simulink model "DR18E_Testpult"  (R2017a)
settings: Solver=ode1  StartTime=0.0  StopTime=Inf  FixedStep=0.001  RelTol=1e-3
PostLoadFcn:
  | , if any(exist('dsrtsu_mdlpostloadfcn', 'file') == [2, 3, 6]), try dsrtsu_mdlpostloadfcn('Execute', bdroot); catch fprintf('Error in PostLoadFcn (dsrtsu_mdlpostloadfcn) for model "%s":\n %s\n', bdroot, lasterr); end, end,
model workspace: external: MATLAB File C:\Users\DeltaRacing\Documents\dSPACE\MABX_DR18E\Model\DR18E_MABX_Parameter.m (data not in the file)
values from neighbouring files (symbols this model uses):
  am = 1/Ts    (= 1)    [DR18E_MABX_Parameter.m]
  bm = K/Ts    (= 0.05)    [DR18E_MABX_Parameter.m]
  cf = 41350    [DR18E_MABX_Parameter.m]
  cr = 41350    [DR18E_MABX_Parameter.m]
  Derating_HV_Battery_Kapa = 1    [DR18E_MABX_Parameter.m]
  Derating_Start_km = 16    [DR18E_MABX_Parameter.m]
  Drive_Mode = 0    [DR18E_MABX_Parameter.m]
  g = 1    [DR18E_MABX_Parameter.m]
  Gas_Modus = 2    [DR18E_MABX_Parameter.m]
  HV_Power_max = 80    [DR18E_MABX_Parameter.m]
  i_Getriebe = 3.3    [DR18E_MABX_Parameter.m]
  i_Lenkgetriebe = 4.32    [DR18E_MABX_Parameter.m]
  K_SET = 1    [DR18E_MABX_Parameter.m]
  Kapazitaet_HV_Battery_kWh = 6.6    [DR18E_MABX_Parameter.m]
  KW_T_Soll = 37    [DR18E_MABX_Parameter.m]
  lf = 1.2    [DR18E_MABX_Parameter.m]
  lr = 1.15    [DR18E_MABX_Parameter.m]
  m = 310    [DR18E_MABX_Parameter.m]
  M_max = 150    [DR18E_MABX_Parameter.m]
  Power_Limit_onoff = 0    [DR18E_MABX_Parameter.m]
  Reifenradius = 0.2351    [DR18E_MABX_Parameter.m]
  Strecke_Endu_km = 22    [DR18E_MABX_Parameter.m]
  TC_Decr_Gas = 0.00005    (= 5e-05)    [DR18E_MABX_Parameter.m]
  TC_Derivative = 0.4    [DR18E_MABX_Parameter.m]
  TC_Incr_Gas = 0.005    [DR18E_MABX_Parameter.m]
  TC_On = 0    [DR18E_MABX_Parameter.m]
  TC_Relay_Off = 0.065    [DR18E_MABX_Parameter.m]
  TC_Relay_On = 0.07    [DR18E_MABX_Parameter.m]
  TV_Mode = 2    [DR18E_MABX_Parameter.m]
  TV_On = 0    [DR18E_MABX_Parameter.m]
  TV_Override = 1    [DR18E_MABX_Parameter.m]
  y = 0.8    [DR18E_MABX_Parameter.m]
undefined symbols (not defined in the file or in its folder): D, DiscIntNeverNeededParam, I, K_OL, P
libraries: simulink x288, rtican x105, rtiusbflightreclib x40, rti1401lib_dio_type3 x10, simulink_extras x10, rti1401lib_adc_type4 x8, rti1401lib_II_base x7
(part 25 of 28)

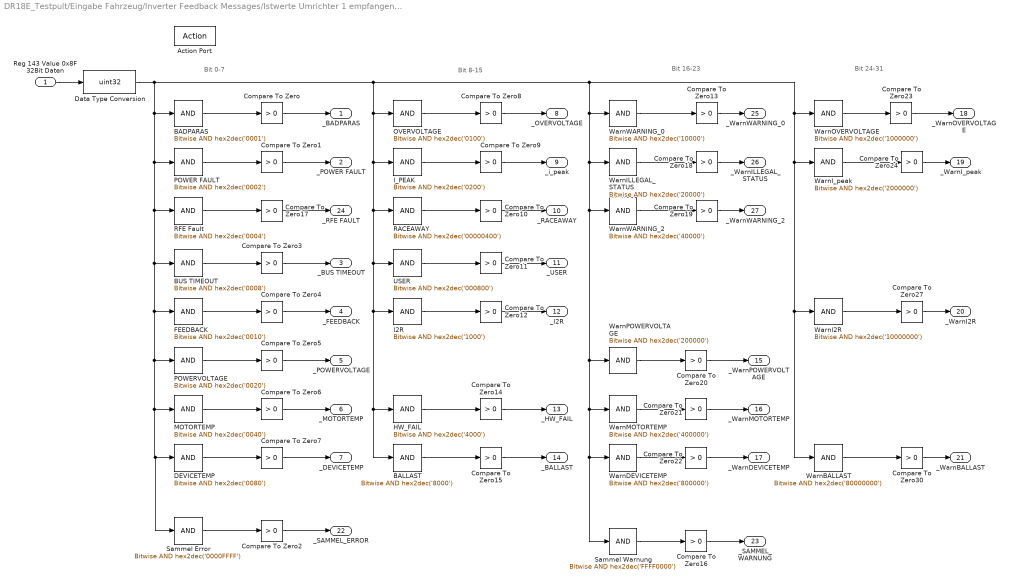
== system DR18E_Testpult/Eingabe Fahrzeug/Inverter Feedback Messages/Istwerte Umrichter 1 empfangen /Reg ID: 0x8F ERROR//Warning Register Auswertung1 ==
  note: Bit 0-7
  note: Bit 8-15
  note: Bit 16-23
  note: Bit 24-31
  Reg 143 Value 0x8F 32Bit Daten : Inport
  Action Port : ActionPort  ActionType=case
  BADPARAS : simulink/Logic and Bit Operations/Bitwise Operator  logicop=AND  UseBitMask=on  BitMask=hex2dec('0001')  BitMaskRealWorld=Stored Integer
  BALLAST : simulink/Logic and Bit Operations/Bitwise Operator  logicop=AND  UseBitMask=on  BitMask=hex2dec('8000')  BitMaskRealWorld=Stored Integer
  BUS TIMEOUT : simulink/Logic and Bit Operations/Bitwise Operator  logicop=AND  UseBitMask=on  BitMask=hex2dec('0008')  BitMaskRealWorld=Stored Integer
  Compare To Zero{,1..24,27,30} (27 alike) : simulink/Logic and Bit Operations/Compare To Zero  relop=>  OutDataTypeStr=boolean
  DEVICETEMP : simulink/Logic and Bit Operations/Bitwise Operator  logicop=AND  UseBitMask=on  BitMask=hex2dec('0080')  BitMaskRealWorld=Stored Integer
  Data Type Conversion : DataTypeConversion  OutDataTypeStr=uint32
  FEEDBACK : simulink/Logic and Bit Operations/Bitwise Operator  logicop=AND  UseBitMask=on  BitMask=hex2dec('0010')  BitMaskRealWorld=Stored Integer
  HW_FAIL : simulink/Logic and Bit Operations/Bitwise Operator  logicop=AND  UseBitMask=on  BitMask=hex2dec('4000')  BitMaskRealWorld=Stored Integer
  I2R : simulink/Logic and Bit Operations/Bitwise Operator  logicop=AND  UseBitMask=on  BitMask=hex2dec('1000')  BitMaskRealWorld=Stored Integer
  I_PEAK : simulink/Logic and Bit Operations/Bitwise Operator  logicop=AND  UseBitMask=on  BitMask=hex2dec('0200')  BitMaskRealWorld=Stored Integer
  MOTORTEMP : simulink/Logic and Bit Operations/Bitwise Operator  logicop=AND  UseBitMask=on  BitMask=hex2dec('0040')  BitMaskRealWorld=Stored Integer
  OVERVOLTAGE : simulink/Logic and Bit Operations/Bitwise Operator  logicop=AND  UseBitMask=on  BitMask=hex2dec('0100')  BitMaskRealWorld=Stored Integer
  POWER FAULT : simulink/Logic and Bit Operations/Bitwise Operator  logicop=AND  UseBitMask=on  BitMask=hex2dec('0002')  BitMaskRealWorld=Stored Integer
  POWERVOLTAGE : simulink/Logic and Bit Operations/Bitwise Operator  logicop=AND  UseBitMask=on  BitMask=hex2dec('0020')  BitMaskRealWorld=Stored Integer
  RACEAWAY : simulink/Logic and Bit Operations/Bitwise Operator  logicop=AND  UseBitMask=on  BitMask=hex2dec('00000400')  BitMaskRealWorld=Stored Integer
  RFE Fault : simulink/Logic and Bit Operations/Bitwise Operator  logicop=AND  UseBitMask=on  BitMask=hex2dec('0004')  BitMaskRealWorld=Stored Integer
  Sammel Error : simulink/Logic and Bit Operations/Bitwise Operator  logicop=AND  UseBitMask=on  BitMask=hex2dec('0000FFFF')  BitMaskRealWorld=Stored Integer
  Sammel Warnung : simulink/Logic and Bit Operations/Bitwise Operator  logicop=AND  UseBitMask=on  BitMask=hex2dec('FFFF0000')  BitMaskRealWorld=Stored Integer
  USER : simulink/Logic and Bit Operations/Bitwise Operator  logicop=AND  UseBitMask=on  BitMask=hex2dec('000800')  BitMaskRealWorld=Stored Integer
  WarnBALLAST : simulink/Logic and Bit Operations/Bitwise Operator  logicop=AND  UseBitMask=on  BitMask=hex2dec('80000000')  BitMaskRealWorld=Stored Integer
  WarnDEVICETEMP : simulink/Logic and Bit Operations/Bitwise Operator  logicop=AND  UseBitMask=on  BitMask=hex2dec('800000')  BitMaskRealWorld=Stored Integer
  WarnI2R : simulink/Logic and Bit Operations/Bitwise Operator  logicop=AND  UseBitMask=on  BitMask=hex2dec('10000000')  BitMaskRealWorld=Stored Integer
  WarnILLEGAL_STATUS : simulink/Logic and Bit Operations/Bitwise Operator  logicop=AND  UseBitMask=on  BitMask=hex2dec('20000')  BitMaskRealWorld=Stored Integer
  WarnI_peak : simulink/Logic and Bit Operations/Bitwise Operator  logicop=AND  UseBitMask=on  BitMask=hex2dec('2000000')  BitMaskRealWorld=Stored Integer
  WarnMOTORTEMP : simulink/Logic and Bit Operations/Bitwise Operator  logicop=AND  UseBitMask=on  BitMask=hex2dec('400000')  BitMaskRealWorld=Stored Integer
  WarnOVERVOLTAGE : simulink/Logic and Bit Operations/Bitwise Operator  logicop=AND  UseBitMask=on  BitMask=hex2dec('1000000')  BitMaskRealWorld=Stored Integer
  WarnPOWERVOLTAGE : simulink/Logic and Bit Operations/Bitwise Operator  logicop=AND  UseBitMask=on  BitMask=hex2dec('200000')  BitMaskRealWorld=Stored Integer
  WarnWARNING_0 : simulink/Logic and Bit Operations/Bitwise Operator  logicop=AND  UseBitMask=on  BitMask=hex2dec('10000')  BitMaskRealWorld=Stored Integer
  WarnWARNING_2 : simulink/Logic and Bit Operations/Bitwise Operator  logicop=AND  UseBitMask=on  BitMask=hex2dec('40000')  BitMaskRealWorld=Stored Integer
  _BADPARAS : Outport
  _POWER FAULT : Outport  Port=2
  _BUS TIMEOUT : Outport  Port=3
  _FEEDBACK : Outport  Port=4
  _POWERVOLTAGE : Outport  Port=5
  _MOTORTEMP : Outport  Port=6
  _DEVICETEMP : Outport  Port=7
  _OVERVOLTAGE : Outport  Port=8
  _i_peak : Outport  Port=9
  _RACEAWAY : Outport  Port=10
  _USER : Outport  Port=11
  _I2R : Outport  Port=12
  _HW_FAIL : Outport  Port=13
  _BALLAST : Outport  Port=14
  _WarnPOWERVOLTAGE : Outport  Port=15
  _WarnMOTORTEMP : Outport  Port=16
  _WarnDEVICETEMP : Outport  Port=17
  _WarnOVERVOLTAGE : Outport  Port=18
  _WarnI_peak : Outport  Port=19
  _WarnI2R : Outport  Port=20
  _WarnBALLAST : Outport  Port=21
  _SAMMEL_ERROR : Outport  Port=22
  _SAMMEL_WARNUNG : Outport  Port=23
  _RFE FAULT : Outport  Port=24
  _WarnWARNING_0 : Outport  Port=25
  _WarnILLEGAL_STATUS : Outport  Port=26
  _WarnWARNING_2 : Outport  Port=27
  wires:
  Compare To Zero16/1 -> _SAMMEL_WARNUNG/1
  Sammel Warnung/1 -> Compare To Zero16/1
  Compare To Zero2/1 -> _SAMMEL_ERROR/1
  Sammel Error/1 -> Compare To Zero2/1
  Compare To Zero30/1 -> _WarnBALLAST/1
  Compare To Zero27/1 -> _WarnI2R/1
  Reg 143 Value 0x8F 32Bit Daten/1 -> Data Type Conversion/1
  WarnBALLAST/1 -> Compare To Zero30/1
  WarnI2R/1 -> Compare To Zero27/1
  Compare To Zero24/1 -> _WarnI_peak/1
  WarnI_peak/1 -> Compare To Zero24/1
  Compare To Zero23/1 -> _WarnOVERVOLTAGE/1
  Compare To Zero22/1 -> _WarnDEVICETEMP/1
  Compare To Zero21/1 -> _WarnMOTORTEMP/1
  Compare To Zero20/1 -> _WarnPOWERVOLTAGE/1
  WarnOVERVOLTAGE/1 -> Compare To Zero23/1
  WarnDEVICETEMP/1 -> Compare To Zero22/1
  WarnMOTORTEMP/1 -> Compare To Zero21/1
  WarnPOWERVOLTAGE/1 -> Compare To Zero20/1
  Compare To Zero15/1 -> _BALLAST/1
  Compare To Zero14/1 -> _HW_FAIL/1
  Compare To Zero12/1 -> _I2R/1
  Compare To Zero11/1 -> _USER/1
  Compare To Zero10/1 -> _RACEAWAY/1
  Compare To Zero9/1 -> _i_peak/1
  Compare To Zero8/1 -> _OVERVOLTAGE/1
  BALLAST/1 -> Compare To Zero15/1
  HW_FAIL/1 -> Compare To Zero14/1
  I2R/1 -> Compare To Zero12/1
  USER/1 -> Compare To Zero11/1
  RACEAWAY/1 -> Compare To Zero10/1
  I_PEAK/1 -> Compare To Zero9/1
  OVERVOLTAGE/1 -> Compare To Zero8/1
  Compare To Zero7/1 -> _DEVICETEMP/1
  Compare To Zero6/1 -> _MOTORTEMP/1
  Compare To Zero5/1 -> _POWERVOLTAGE/1
  Compare To Zero4/1 -> _FEEDBACK/1
  Compare To Zero3/1 -> _BUS TIMEOUT/1
  Compare To Zero1/1 -> _POWER FAULT/1
  Compare To Zero/1 -> _BADPARAS/1
  DEVICETEMP/1 -> Compare To Zero7/1
  MOTORTEMP/1 -> Compare To Zero6/1
  POWERVOLTAGE/1 -> Compare To Zero5/1
  FEEDBACK/1 -> Compare To Zero4/1
  BUS TIMEOUT/1 -> Compare To Zero3/1
  POWER FAULT/1 -> Compare To Zero1/1
  BADPARAS/1 -> Compare To Zero/1
  Compare To Zero17/1 -> _RFE FAULT/1
  Data Type Conversion/1 -> BADPARAS/1, RFE Fault/1, BUS TIMEOUT/1, FEEDBACK/1, POWERVOLTAGE/1, MOTORTEMP/1, DEVICETEMP/1, Sammel Error/1, POWER FAULT/1, OVERVOLTAGE/1, RACEAWAY/1, USER/1, I2R/1, HW_FAIL/1, BALLAST/1, I_PEAK/1, WarnWARNING_0/1, WarnILLEGAL_STATUS/1, WarnWARNING_2/1, WarnMOTORTEMP/1, WarnDEVICETEMP/1, Sammel Warnung/1, WarnPOWERVOLTAGE/1, WarnOVERVOLTAGE/1, WarnI_peak/1, WarnI2R/1, WarnBALLAST/1
  RFE Fault/1 -> Compare To Zero17/1
  Compare To Zero13/1 -> _WarnWARNING_0/1
  WarnWARNING_0/1 -> Compare To Zero13/1
  Compare To Zero18/1 -> _WarnILLEGAL_STATUS/1
  WarnILLEGAL_STATUS/1 -> Compare To Zero18/1
  Compare To Zero19/1 -> _WarnWARNING_2/1
  WarnWARNING_2/1 -> Compare To Zero19/1

== system DR18E_Testpult/Eingabe Fahrzeug/Inverter Feedback Messages/Istwerte Umrichter 1 empfangen /Sender OK Detection ==
  note: This subsystem implements the surveying of the sender corresponding to the RX message.
      |
      | If for 6 consecutive execution steps no message is received it is considered that the sender is no
      | longer alive or in serious trouble and the 'RX Warn' output is set to 1.
      |
      | Also, the message is expected to be received every 50 ms approximatively. If this condition is not
      | met 6 times consecutively the 'RX Warn' output is set to 1.
  RX status : Inport
  RX delta time : Inport  Port=2
  AND : Logic
  Delta time limit : Constant  Value=0.055
  Delta time limit exceeded : RelationalOperator  RndMeth=Nearest  InputSameDT=on
  Mem{1..5} (5 alike) : Memory
  New data : RelationalOperator  Operator===  RndMeth=Nearest  InputSameDT=on
  New data value : Constant
  No data : RelationalOperator  Operator===  RndMeth=Nearest  InputSameDT=on
  No data value : Constant  Value=0
  OR : Logic  Operator=OR
  Warn : Logic  Inputs=6
  RX Warn : Outport
  wires:
  New data value/1 -> New data/2
  Delta time limit exceeded/1 -> AND/2
  Delta time limit/1 -> Delta time limit exceeded/2
  RX delta time/1 -> Delta time limit exceeded/1
  New data/1 -> AND/1
  AND/1 -> OR/2
  No data value/1 -> No data/2
  No data/1 -> OR/1
  RX status/1 -> No data/1, New data/1
  OR/1 -> Mem1/1, Warn/1
  Mem1/1 -> Mem2/1, Warn/2
  Mem2/1 -> Mem3/1, Warn/3
  Mem3/1 -> Mem4/1, Warn/4
  Warn/1 -> RX Warn/1
  Mem4/1 -> Mem5/1, Warn/5
  Mem5/1 -> Warn/6

== system DR18E_Testpult/Eingabe Fahrzeug/Inverter Feedback Messages/Istwerte Umrichter 1 empfangen /Strom ==
  In2 : Inport
  Action Port : ActionPort  ActionType=case
  Constant2 : Constant  Value=560
  Data Type Conversion4 : DataTypeConversion  OutDataTypeStr=int16
  Divide2 : Product  Inputs=*/
  Drehmoment / Strangstrom in Nm/Arms : Gain  Gain=0.75
  Gain2 : Gain  Gain=200
  Strangstrom I_rms in A U1 : Outport
  Drehmoment M in Nm U1 : Outport  Port=2
  wires:
  In2/1 -> Data Type Conversion4/1
  Gain2/1 -> Divide2/1
  Constant2/1 -> Divide2/2
  Drehmoment / Strangstrom in Nm/Arms/1 -> Drehmoment M in Nm U1/1
  Data Type Conversion4/1 -> Gain2/1
  Divide2/1 -> Drehmoment / Strangstrom in Nm/Arms/1, Strangstrom I_rms in A U1/1

== system DR18E_Testpult/Eingabe Fahrzeug/Inverter Feedback Messages/Istwerte Umrichter 1 empfangen /U_DC ==
  In1 : Inport
  Action Port : ActionPort  ActionType=case
  Umrechnung Register--> Spannung Manual BAMOCAR PG D3 S. 47 : Gain  Gain=1/31.499
  U_DC : Outport
  wires:
  In1/1 -> Umrechnung Register--> Spannung Manual BAMOCAR PG D3 S. 47/1  "Wert"
  Umrechnung Register--> Spannung Manual BAMOCAR PG D3 S. 47/1 -> U_DC/1

== system DR18E_Testpult/Eingabe Fahrzeug/Inverter Feedback Messages/Istwerte Umrichter 1 empfangen /Wirkstrom Iq ==
  In1 : Inport
  Action Port : ActionPort  ActionType=case
  Constant2 : Constant  Value=560
  Data Type Conversion1 : DataTypeConversion  OutDataTypeStr=int16
  Divide2 : Product  Inputs=*/
  Faktor 3/2 : Constant  Value=1.5
  Gain3 : Gain  Gain=200
  Polpaarzahl p : Constant  Value=10
  Product : Product  Inputs=4
  magnertischer Fluß Psi in Vs : Constant  Value=0.053
  Wirkstrom Iq in A U1 : Outport
  Drehmoment in Nm aus Iq U1 : Outport  Port=2
  wires:
  Divide2/1 -> Wirkstrom Iq in A U1/1, Product/1
  In1/1 -> Data Type Conversion1/1
  Gain3/1 -> Divide2/1
  Constant2/1 -> Divide2/2
  Polpaarzahl p/1 -> Product/2
  Faktor 3/2/1 -> Product/3
  magnertischer Fluß Psi in Vs/1 -> Product/4
  Product/1 -> Drehmoment in Nm aus Iq U1/1
  Data Type Conversion1/1 -> Gain3/1

== system DR18E_Testpult/Eingabe Fahrzeug/Inverter Feedback Messages/Istwerte Umrichter 2 empfangen/Drehzahl ==
  CAN Value : Inport
  M_Mot : Inport  Port=2
  Action Port : ActionPort  ActionType=case
  2*p / 60i : Gain  Gain=1.8*6.283185 / 60
  Constant1 : Constant  Value=-1
  Data Type Conversion : DataTypeConversion  OutDataTypeStr=int16
  Data Type Conversion1 : DataTypeConversion  OutDataTypeStr=double
  PT1 Discrete2 : Subsystem
  Product : Product
  Skalierung Drehzahl : Subsystem  TreatAsAtomicUnit=on
  TFilterDrehzahl : Constant  Value=0.01
  Drehzahl in 1/min U1 : Outport
  Motorleistung in W U1 : Outport  Port=2
  wires:
  CAN Value/1 -> Data Type Conversion/1
  PT1 Discrete2/1(y) -> Drehzahl in 1/min U1/1, Product/1
  Data Type Conversion/1 -> Data Type Conversion1/1
  Product/1 -> 2*p / 60i/1
  M_Mot/1 -> Product/2
  2*p / 60i/1 -> Motorleistung in W U1/1
  Constant1/1 -> PT1 Discrete2/2(K)
  TFilterDrehzahl/1 -> PT1 Discrete2/3(T)
  Skalierung Drehzahl/1(Out1) -> PT1 Discrete2/1(u)
  Data Type Conversion1/1 -> Skalierung Drehzahl/1(In1)

== system DR18E_Testpult/Eingabe Fahrzeug/Inverter Feedback Messages/Istwerte Umrichter 2 empfangen/FlightRecorder2 ==
  In1 : Inport
  Data Type Conversion : DataTypeConversion
  Gain : Gain
  USB_FLIGHT_REC_BL1 : rtiusbflightreclib/USB_FLIGHT_REC_BL1  VarName=MMotR_Ist  DataType=Single  SampleTime=-1  TLCFileName=rtiusbflightrecwrite  Reserved1=[]  Reserved2=[]  Reserved3=[]  Reserved4=[]  DSProperties=struct('RTI',struct('Version',uint32(3),'BlockType',struct('isSLSource',uint8(0),'isSLSink',uint8(1),'isHWSource',uint8(0),'isHWSink',uint8(0),'isSetup',uint8(0),'isInline',uint8(1),'isNonInline',uint8(0),'isInterrupt',uint8(0),'isChannelwise',uint8(0)),'IOBoardType',{{'DSUSB','FLIGHTREC'}},'UnitType','FLIGHTREC','Identifier','WRITE','DialogType','SL','BlockSet','RTIUSBFLIGHTREC','SlaveProcessor','NONE'))  RTIBlockInterface=struct('InputPortsActive',1,'InputPortsWidth',int32(1),'InputPortsDataType',{{'SS_SINGLE'}},'BlockDisplay',{{['Write to\nUSB Flight Recorder'],'center'}},'IconTransparency','off','InitLevel',3,'BlockName',struct('Token',{{'USB_FLIGHT_REC_BL1'}}),'MaskDescription',['Write input to the Flight Recorder. Recorded data can be referenced by the specified variable.'],'SampleTime',{{-1}})  RTIBlockParameters=struct('VarName',{{'MMotR_Ist','OFF',[]}},'DataType',{{'Single','OFF',[]}},'SampleTime',{{-1,'OFF',[]}},'TLCFileName',{{'rtiusbflightrecwrite','OFF',[]}})  RTISFcnParameters=struct('VarName','char','DataType','char','SampleTime','double','TLCFileName','char')  RTIBlockParaDefault=struct('VarName','Var1','DataType','Single','SampleTime',-1,'TLCFileName','rtiusbflightrecwrite')
      settings: SourceProductName=dSPACE RTI USB Flight Rec Blockset
  wires:
  Data Type Conversion/1 -> USB_FLIGHT_REC_BL1/1
  In1/1 -> Gain/1
  Gain/1 -> Data Type Conversion/1

== system DR18E_Testpult/Eingabe Fahrzeug/Inverter Feedback Messages/Istwerte Umrichter 2 empfangen/Inverter_Temp ==
  In1 : Inport
  Action Port : ActionPort  ActionType=case
  "BAMOCAR PG D3 Manual S. 48 " : Lookup_n-D  NumberOfTableDimensions=1  BreakpointsForDimension1=[17151,17400,17688,18017,18387,18797,19247,19733,20250,20793,21357,21933,22515,23097,23671,24232,24775,25296,25792,26261,26702]  Table=[0,5,10,15,20,25,30,35,40,45,50,55,60,65,70,75,80,85,90,95,100]  RndMeth=Simplest  InputSameDT=on
  Inverter_Temp : Outport
  wires:
  In1/1 -> "BAMOCAR PG D3 Manual S. 48 "/1  "Wert"
  "BAMOCAR PG D3 Manual S. 48 "/1 -> Inverter_Temp/1

== system DR18E_Testpult/Eingabe Fahrzeug/Inverter Feedback Messages/Istwerte Umrichter 2 empfangen/Motortemperatur ==
  In1 : Inport
  Action Port : ActionPort  ActionType=case
  Constant2 : Constant  Value=37175
  Divide : Product  Inputs=*/
  Gain : Gain  Gain=4700
  Subtract : Sum  Inputs=+-
  Temp. corresponding resistance : Lookup_n-D  NumberOfTableDimensions=1  BreakpointsForDimension1=[1030,1135,1247,1367,1495,1630,1772,1922,2000,2080,2245,2417,2597,2785,2980,3182,3392,3607,3817,3915,4008,4166,4280]  IndexSearchMethod=Linear search  Table=[-50,-40,-30,-20,-10,0,10,20,25,30,40,50,60,70,80,90,100,110,120,125,130,140,150]  RndMeth=Simplest  InputSameDT=on
  Motor1_Temp : Outport
  "Motor1_R " : Outport  Port=2
  wires:
  Gain/1 -> Divide/1
  Subtract/1 -> Divide/2
  Constant2/1 -> Subtract/1
  In1/1 -> Subtract/2, Gain/1  "Wert"
  Divide/1 -> "Motor1_R "/1, Temp. corresponding resistance/1
  Temp. corresponding resistance/1 -> Motor1_Temp/1

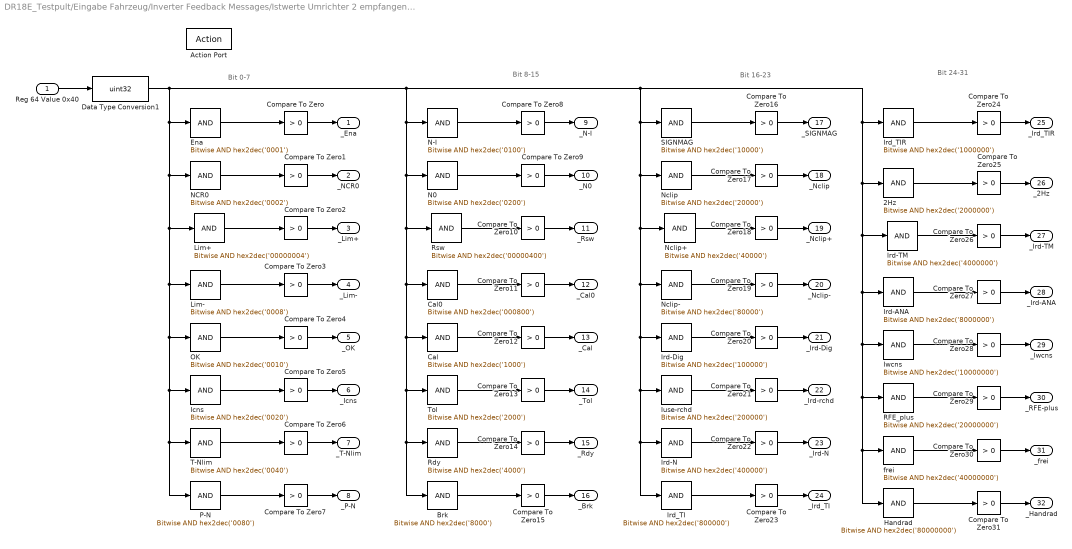
== system DR18E_Testpult/Eingabe Fahrzeug/Inverter Feedback Messages/Istwerte Umrichter 2 empfangen/Red ID 64: Status Register Auswertung ==
  note: Bit 16-23
  note: Bit 24-31
  note: Bit 8-15
  note: Bit 0-7
  Reg 64 Value 0x40 : Inport
  Action Port : ActionPort  ActionType=case
  2Hz : simulink/Logic and Bit Operations/Bitwise Operator  logicop=AND  UseBitMask=on  BitMask=hex2dec('2000000')  BitMaskRealWorld=Stored Integer
  Brk : simulink/Logic and Bit Operations/Bitwise Operator  logicop=AND  UseBitMask=on  BitMask=hex2dec('8000')  BitMaskRealWorld=Stored Integer
  Cal : simulink/Logic and Bit Operations/Bitwise Operator  logicop=AND  UseBitMask=on  BitMask=hex2dec('1000')  BitMaskRealWorld=Stored Integer
  Cal0 : simulink/Logic and Bit Operations/Bitwise Operator  logicop=AND  UseBitMask=on  BitMask=hex2dec('000800')  BitMaskRealWorld=Stored Integer
  Compare To Zero{,1..31} (32 alike) : simulink/Logic and Bit Operations/Compare To Zero  relop=>  OutDataTypeStr=boolean
  Data Type Conversion1 : DataTypeConversion  OutDataTypeStr=uint32
  Ena : simulink/Logic and Bit Operations/Bitwise Operator  logicop=AND  UseBitMask=on  BitMask=hex2dec('0001')  BitMaskRealWorld=Stored Integer
  Handrad : simulink/Logic and Bit Operations/Bitwise Operator  logicop=AND  UseBitMask=on  BitMask=hex2dec('80000000')  BitMaskRealWorld=Stored Integer
  Icns : simulink/Logic and Bit Operations/Bitwise Operator  logicop=AND  UseBitMask=on  BitMask=hex2dec('0020')  BitMaskRealWorld=Stored Integer
  Ird-ANA : simulink/Logic and Bit Operations/Bitwise Operator  logicop=AND  UseBitMask=on  BitMask=hex2dec('8000000')  BitMaskRealWorld=Stored Integer
  Ird-Dig : simulink/Logic and Bit Operations/Bitwise Operator  logicop=AND  UseBitMask=on  BitMask=hex2dec('100000')  BitMaskRealWorld=Stored Integer
  Ird-N : simulink/Logic and Bit Operations/Bitwise Operator  logicop=AND  UseBitMask=on  BitMask=hex2dec('400000')  BitMaskRealWorld=Stored Integer
  Ird-TM : simulink/Logic and Bit Operations/Bitwise Operator  logicop=AND  UseBitMask=on  BitMask=hex2dec('4000000')  BitMaskRealWorld=Stored Integer
  Ird_TI : simulink/Logic and Bit Operations/Bitwise Operator  logicop=AND  UseBitMask=on  BitMask=hex2dec('800000')  BitMaskRealWorld=Stored Integer
  Ird_TIR : simulink/Logic and Bit Operations/Bitwise Operator  logicop=AND  UseBitMask=on  BitMask=hex2dec('1000000')  BitMaskRealWorld=Stored Integer
  Iuse-rchd : simulink/Logic and Bit Operations/Bitwise Operator  logicop=AND  UseBitMask=on  BitMask=hex2dec('200000')  BitMaskRealWorld=Stored Integer
  Iwcns : simulink/Logic and Bit Operations/Bitwise Operator  logicop=AND  UseBitMask=on  BitMask=hex2dec('10000000')  BitMaskRealWorld=Stored Integer
  Lim+ : simulink/Logic and Bit Operations/Bitwise Operator  logicop=AND  UseBitMask=on  BitMask=hex2dec('00000004')  BitMaskRealWorld=Stored Integer
  Lim- : simulink/Logic and Bit Operations/Bitwise Operator  logicop=AND  UseBitMask=on  BitMask=hex2dec('0008')  BitMaskRealWorld=Stored Integer
  N-I : simulink/Logic and Bit Operations/Bitwise Operator  logicop=AND  UseBitMask=on  BitMask=hex2dec('0100')  BitMaskRealWorld=Stored Integer
  N0 : simulink/Logic and Bit Operations/Bitwise Operator  logicop=AND  UseBitMask=on  BitMask=hex2dec('0200')  BitMaskRealWorld=Stored Integer
  NCR0 : simulink/Logic and Bit Operations/Bitwise Operator  logicop=AND  UseBitMask=on  BitMask=hex2dec('0002')  BitMaskRealWorld=Stored Integer
  Nclip : simulink/Logic and Bit Operations/Bitwise Operator  logicop=AND  UseBitMask=on  BitMask=hex2dec('20000')  BitMaskRealWorld=Stored Integer
  Nclip+ : simulink/Logic and Bit Operations/Bitwise Operator  logicop=AND  UseBitMask=on  BitMask=hex2dec('40000')  BitMaskRealWorld=Stored Integer
  Nclip- : simulink/Logic and Bit Operations/Bitwise Operator  logicop=AND  UseBitMask=on  BitMask=hex2dec('80000')  BitMaskRealWorld=Stored Integer
  OK : simulink/Logic and Bit Operations/Bitwise Operator  logicop=AND  UseBitMask=on  BitMask=hex2dec('0010')  BitMaskRealWorld=Stored Integer
  P-N : simulink/Logic and Bit Operations/Bitwise Operator  logicop=AND  UseBitMask=on  BitMask=hex2dec('0080')  BitMaskRealWorld=Stored Integer
  RFE_plus : simulink/Logic and Bit Operations/Bitwise Operator  logicop=AND  UseBitMask=on  BitMask=hex2dec('20000000')  BitMaskRealWorld=Stored Integer
  Rdy : simulink/Logic and Bit Operations/Bitwise Operator  logicop=AND  UseBitMask=on  BitMask=hex2dec('4000')  BitMaskRealWorld=Stored Integer
  Rsw : simulink/Logic and Bit Operations/Bitwise Operator  logicop=AND  UseBitMask=on  BitMask=hex2dec('00000400')  BitMaskRealWorld=Stored Integer
  SIGNMAG : simulink/Logic and Bit Operations/Bitwise Operator  logicop=AND  UseBitMask=on  BitMask=hex2dec('10000')  BitMaskRealWorld=Stored Integer
  T-Nlim : simulink/Logic and Bit Operations/Bitwise Operator  logicop=AND  UseBitMask=on  BitMask=hex2dec('0040')  BitMaskRealWorld=Stored Integer
  Tol : simulink/Logic and Bit Operations/Bitwise Operator  logicop=AND  UseBitMask=on  BitMask=hex2dec('2000')  BitMaskRealWorld=Stored Integer
  frei : simulink/Logic and Bit Operations/Bitwise Operator  logicop=AND  UseBitMask=on  BitMask=hex2dec('40000000')  BitMaskRealWorld=Stored Integer
  _Ena : Outport
  _NCR0 : Outport  Port=2
  _Lim+ : Outport  Port=3
  _Lim- : Outport  Port=4
  _OK : Outport  Port=5
  _Icns : Outport  Port=6
  _T-Nlim : Outport  Port=7
  _P-N : Outport  Port=8
  _N-I : Outport  Port=9
  _N0 : Outport  Port=10
  _Rsw : Outport  Port=11
  _Cal0 : Outport  Port=12
  _Cal : Outport  Port=13
  _Tol : Outport  Port=14
  _Rdy : Outport  Port=15
  _Brk : Outport  Port=16
  _SIGNMAG : Outport  Port=17
  _Nclip : Outport  Port=18
  _Nclip+ : Outport  Port=19
  _Nclip- : Outport  Port=20
  _Ird-Dig : Outport  Port=21
  _Ird-rchd : Outport  Port=22
  _Ird-N : Outport  Port=23
  _Ird_TI : Outport  Port=24
  _Ird_TIR : Outport  Port=25
  _2Hz : Outport  Port=26
  _Ird-TM : Outport  Port=27
  _Ird-ANA : Outport  Port=28
  _Iwcns : Outport  Port=29
  _RFE-plus : Outport  Port=30
  _frei : Outport  Port=31
  _Handrad : Outport  Port=32
  wires:
  Reg 64 Value 0x40/1 -> Data Type Conversion1/1
  2Hz/1 -> Compare To Zero25/1
  Iwcns/1 -> Compare To Zero28/1
  Compare To Zero25/1 -> _2Hz/1
  Compare To Zero29/1 -> _RFE-plus/1
  Ird-ANA/1 -> Compare To Zero27/1
  Compare To Zero26/1 -> _Ird-TM/1
  Handrad/1 -> Compare To Zero31/1
  RFE_plus/1 -> Compare To Zero29/1
  Compare To Zero27/1 -> _Ird-ANA/1
  Ird-TM/1 -> Compare To Zero26/1
  frei/1 -> Compare To Zero30/1
  Compare To Zero28/1 -> _Iwcns/1
  Tol/1 -> Compare To Zero13/1
  Nclip+/1 -> Compare To Zero18/1
  Compare To Zero17/1 -> _Nclip/1
  Compare To Zero16/1 -> _SIGNMAG/1
  Ird-N/1 -> Compare To Zero22/1
  Ird_TI/1 -> Compare To Zero23/1
  Compare To Zero20/1 -> _Ird-Dig/1
  Lim+/1 -> Compare To Zero2/1
  Nclip-/1 -> Compare To Zero19/1
  SIGNMAG/1 -> Compare To Zero16/1
  Compare To Zero12/1 -> _Cal/1
  Compare To Zero3/1 -> _Lim-/1
  Compare To Zero2/1 -> _Lim+/1
  Compare To Zero8/1 -> _N-I/1
  N-I/1 -> Compare To Zero8/1
  Brk/1 -> Compare To Zero15/1
  Compare To Zero/1 -> _Ena/1
  Compare To Zero6/1 -> _T-Nlim/1
  Compare To Zero1/1 -> _NCR0/1
  P-N/1 -> Compare To Zero7/1
  Icns/1 -> Compare To Zero5/1
  T-Nlim/1 -> Compare To Zero6/1
  Compare To Zero9/1 -> _N0/1
  Cal/1 -> Compare To Zero12/1
  Rdy/1 -> Compare To Zero14/1
  Compare To Zero5/1 -> _Icns/1
  NCR0/1 -> Compare To Zero1/1
  Ena/1 -> Compare To Zero/1
  Compare To Zero30/1 -> _frei/1
  Iuse-rchd/1 -> Compare To Zero21/1
  Compare To Zero19/1 -> _Nclip-/1
  Compare To Zero23/1 -> _Ird_TI/1
  Ird_TIR/1 -> Compare To Zero24/1
  Compare To Zero31/1 -> _Handrad/1
  Cal0/1 -> Compare To Zero11/1
  Compare To Zero7/1 -> _P-N/1
  Compare To Zero24/1 -> _Ird_TIR/1
  Compare To Zero22/1 -> _Ird-N/1
  Compare To Zero4/1 -> _OK/1
  Compare To Zero10/1 -> _Rsw/1
  Compare To Zero21/1 -> _Ird-rchd/1
  Compare To Zero15/1 -> _Brk/1
  Compare To Zero11/1 -> _Cal0/1
  OK/1 -> Compare To Zero4/1
  Compare To Zero13/1 -> _Tol/1
  Compare To Zero14/1 -> _Rdy/1
  N0/1 -> Compare To Zero9/1
  Ird-Dig/1 -> Compare To Zero20/1
  Lim-/1 -> Compare To Zero3/1
  Compare To Zero18/1 -> _Nclip+/1
  Nclip/1 -> Compare To Zero17/1
  Rsw/1 -> Compare To Zero10/1
  Data Type Conversion1/1 -> 2Hz/1, Handrad/1, frei/1, RFE_plus/1, Iwcns/1, Ird-ANA/1, Ird-TM/1, Ird_TIR/1, Nclip/1, Ird_TI/1, Ird-N/1, Iuse-rchd/1, Ird-Dig/1, Nclip-/1, Nclip+/1, SIGNMAG/1, N0/1, Brk/1, Rdy/1, Tol/1, Cal/1, Cal0/1, Rsw/1, N-I/1, NCR0/1, P-N/1, T-Nlim/1, Icns/1, OK/1, Lim-/1, Lim+/1, Ena/1

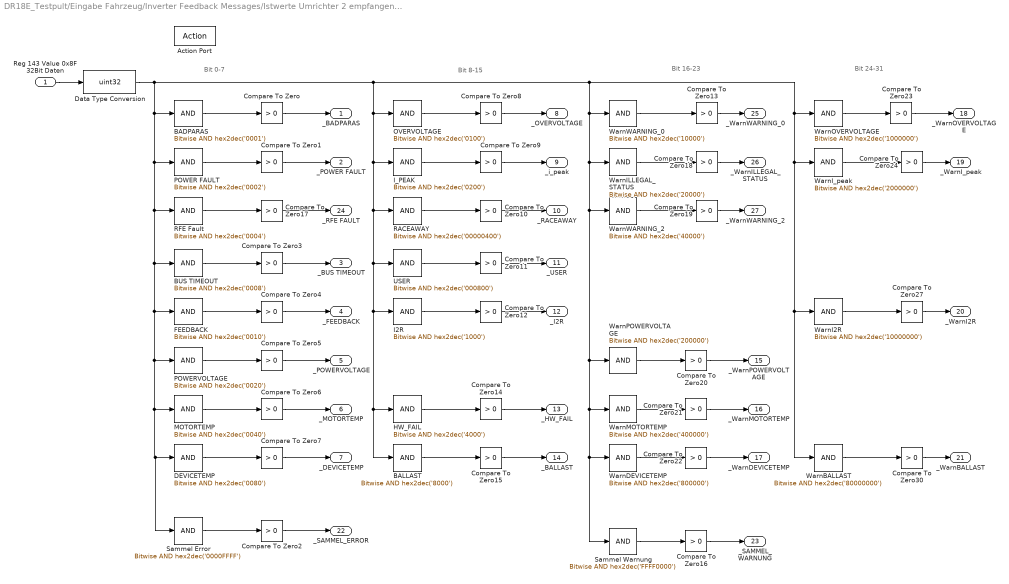
== system DR18E_Testpult/Eingabe Fahrzeug/Inverter Feedback Messages/Istwerte Umrichter 2 empfangen/Reg ID: 0x8F ERROR//Warning Register Auswertung1 ==
  note: Bit 8-15
  note: Bit 0-7
  note: Bit 24-31
  note: Bit 16-23
  Reg 143 Value 0x8F 32Bit Daten : Inport
  Action Port : ActionPort  ActionType=case
  BADPARAS : simulink/Logic and Bit Operations/Bitwise Operator  logicop=AND  UseBitMask=on  BitMask=hex2dec('0001')  BitMaskRealWorld=Stored Integer
  BALLAST : simulink/Logic and Bit Operations/Bitwise Operator  logicop=AND  UseBitMask=on  BitMask=hex2dec('8000')  BitMaskRealWorld=Stored Integer
  BUS TIMEOUT : simulink/Logic and Bit Operations/Bitwise Operator  logicop=AND  UseBitMask=on  BitMask=hex2dec('0008')  BitMaskRealWorld=Stored Integer
  Compare To Zero{,1..24,27,30} (27 alike) : simulink/Logic and Bit Operations/Compare To Zero  relop=>  OutDataTypeStr=boolean
  DEVICETEMP : simulink/Logic and Bit Operations/Bitwise Operator  logicop=AND  UseBitMask=on  BitMask=hex2dec('0080')  BitMaskRealWorld=Stored Integer
  Data Type Conversion : DataTypeConversion  OutDataTypeStr=uint32
  FEEDBACK : simulink/Logic and Bit Operations/Bitwise Operator  logicop=AND  UseBitMask=on  BitMask=hex2dec('0010')  BitMaskRealWorld=Stored Integer
  HW_FAIL : simulink/Logic and Bit Operations/Bitwise Operator  logicop=AND  UseBitMask=on  BitMask=hex2dec('4000')  BitMaskRealWorld=Stored Integer
  I2R : simulink/Logic and Bit Operations/Bitwise Operator  logicop=AND  UseBitMask=on  BitMask=hex2dec('1000')  BitMaskRealWorld=Stored Integer
  I_PEAK : simulink/Logic and Bit Operations/Bitwise Operator  logicop=AND  UseBitMask=on  BitMask=hex2dec('0200')  BitMaskRealWorld=Stored Integer
  MOTORTEMP : simulink/Logic and Bit Operations/Bitwise Operator  logicop=AND  UseBitMask=on  BitMask=hex2dec('0040')  BitMaskRealWorld=Stored Integer
  OVERVOLTAGE : simulink/Logic and Bit Operations/Bitwise Operator  logicop=AND  UseBitMask=on  BitMask=hex2dec('0100')  BitMaskRealWorld=Stored Integer
  POWER FAULT : simulink/Logic and Bit Operations/Bitwise Operator  logicop=AND  UseBitMask=on  BitMask=hex2dec('0002')  BitMaskRealWorld=Stored Integer
  POWERVOLTAGE : simulink/Logic and Bit Operations/Bitwise Operator  logicop=AND  UseBitMask=on  BitMask=hex2dec('0020')  BitMaskRealWorld=Stored Integer
  RACEAWAY : simulink/Logic and Bit Operations/Bitwise Operator  logicop=AND  UseBitMask=on  BitMask=hex2dec('00000400')  BitMaskRealWorld=Stored Integer
  RFE Fault : simulink/Logic and Bit Operations/Bitwise Operator  logicop=AND  UseBitMask=on  BitMask=hex2dec('0004')  BitMaskRealWorld=Stored Integer
  Sammel Error : simulink/Logic and Bit Operations/Bitwise Operator  logicop=AND  UseBitMask=on  BitMask=hex2dec('0000FFFF')  BitMaskRealWorld=Stored Integer
  Sammel Warnung : simulink/Logic and Bit Operations/Bitwise Operator  logicop=AND  UseBitMask=on  BitMask=hex2dec('FFFF0000')  BitMaskRealWorld=Stored Integer
  USER : simulink/Logic and Bit Operations/Bitwise Operator  logicop=AND  UseBitMask=on  BitMask=hex2dec('000800')  BitMaskRealWorld=Stored Integer
  WarnBALLAST : simulink/Logic and Bit Operations/Bitwise Operator  logicop=AND  UseBitMask=on  BitMask=hex2dec('80000000')  BitMaskRealWorld=Stored Integer
  WarnDEVICETEMP : simulink/Logic and Bit Operations/Bitwise Operator  logicop=AND  UseBitMask=on  BitMask=hex2dec('800000')  BitMaskRealWorld=Stored Integer
  WarnI2R : simulink/Logic and Bit Operations/Bitwise Operator  logicop=AND  UseBitMask=on  BitMask=hex2dec('10000000')  BitMaskRealWorld=Stored Integer
  WarnILLEGAL_STATUS : simulink/Logic and Bit Operations/Bitwise Operator  logicop=AND  UseBitMask=on  BitMask=hex2dec('20000')  BitMaskRealWorld=Stored Integer
  WarnI_peak : simulink/Logic and Bit Operations/Bitwise Operator  logicop=AND  UseBitMask=on  BitMask=hex2dec('2000000')  BitMaskRealWorld=Stored Integer
  WarnMOTORTEMP : simulink/Logic and Bit Operations/Bitwise Operator  logicop=AND  UseBitMask=on  BitMask=hex2dec('400000')  BitMaskRealWorld=Stored Integer
  WarnOVERVOLTAGE : simulink/Logic and Bit Operations/Bitwise Operator  logicop=AND  UseBitMask=on  BitMask=hex2dec('1000000')  BitMaskRealWorld=Stored Integer
  WarnPOWERVOLTAGE : simulink/Logic and Bit Operations/Bitwise Operator  logicop=AND  UseBitMask=on  BitMask=hex2dec('200000')  BitMaskRealWorld=Stored Integer
  WarnWARNING_0 : simulink/Logic and Bit Operations/Bitwise Operator  logicop=AND  UseBitMask=on  BitMask=hex2dec('10000')  BitMaskRealWorld=Stored Integer
  WarnWARNING_2 : simulink/Logic and Bit Operations/Bitwise Operator  logicop=AND  UseBitMask=on  BitMask=hex2dec('40000')  BitMaskRealWorld=Stored Integer
  _BADPARAS : Outport
  _POWER FAULT : Outport  Port=2
  _BUS TIMEOUT : Outport  Port=3
  _FEEDBACK : Outport  Port=4
  _POWERVOLTAGE : Outport  Port=5
  _MOTORTEMP : Outport  Port=6
  _DEVICETEMP : Outport  Port=7
  _OVERVOLTAGE : Outport  Port=8
  _i_peak : Outport  Port=9
  _RACEAWAY : Outport  Port=10
  _USER : Outport  Port=11
  _I2R : Outport  Port=12
  _HW_FAIL : Outport  Port=13
  _BALLAST : Outport  Port=14
  _WarnPOWERVOLTAGE : Outport  Port=15
  _WarnMOTORTEMP : Outport  Port=16
  _WarnDEVICETEMP : Outport  Port=17
  _WarnOVERVOLTAGE : Outport  Port=18
  _WarnI_peak : Outport  Port=19
  _WarnI2R : Outport  Port=20
  _WarnBALLAST : Outport  Port=21
  _SAMMEL_ERROR : Outport  Port=22
  _SAMMEL_WARNUNG : Outport  Port=23
  _RFE FAULT : Outport  Port=24
  _WarnWARNING_0 : Outport  Port=25
  _WarnILLEGAL_STATUS : Outport  Port=26
  _WarnWARNING_2 : Outport  Port=27
  wires:
  Reg 143 Value 0x8F 32Bit Daten/1 -> Data Type Conversion/1
  MOTORTEMP/1 -> Compare To Zero6/1
  BUS TIMEOUT/1 -> Compare To Zero3/1
  Compare To Zero12/1 -> _I2R/1
  FEEDBACK/1 -> Compare To Zero4/1
  HW_FAIL/1 -> Compare To Zero14/1
  BADPARAS/1 -> Compare To Zero/1
  Compare To Zero3/1 -> _BUS TIMEOUT/1
  DEVICETEMP/1 -> Compare To Zero7/1
  Compare To Zero6/1 -> _MOTORTEMP/1
  WarnBALLAST/1 -> Compare To Zero30/1
  RACEAWAY/1 -> Compare To Zero10/1
  Compare To Zero15/1 -> _BALLAST/1
  Compare To Zero5/1 -> _POWERVOLTAGE/1
  OVERVOLTAGE/1 -> Compare To Zero8/1
  Compare To Zero1/1 -> _POWER FAULT/1
  Compare To Zero9/1 -> _i_peak/1
  Compare To Zero4/1 -> _FEEDBACK/1
  Compare To Zero/1 -> _BADPARAS/1
  Compare To Zero10/1 -> _RACEAWAY/1
  I_PEAK/1 -> Compare To Zero9/1
  BALLAST/1 -> Compare To Zero15/1
  USER/1 -> Compare To Zero11/1
  Compare To Zero14/1 -> _HW_FAIL/1
  Compare To Zero8/1 -> _OVERVOLTAGE/1
  Compare To Zero16/1 -> _SAMMEL_WARNUNG/1
  Compare To Zero23/1 -> _WarnOVERVOLTAGE/1
  Compare To Zero11/1 -> _USER/1
  WarnPOWERVOLTAGE/1 -> Compare To Zero20/1
  Compare To Zero27/1 -> _WarnI2R/1
  Compare To Zero2/1 -> _SAMMEL_ERROR/1
  WarnOVERVOLTAGE/1 -> Compare To Zero23/1
  WarnI_peak/1 -> Compare To Zero24/1
  Sammel Warnung/1 -> Compare To Zero16/1
  POWERVOLTAGE/1 -> Compare To Zero5/1
  Compare To Zero7/1 -> _DEVICETEMP/1
  WarnI2R/1 -> Compare To Zero27/1
  POWER FAULT/1 -> Compare To Zero1/1
  WarnMOTORTEMP/1 -> Compare To Zero21/1
  WarnDEVICETEMP/1 -> Compare To Zero22/1
  Compare To Zero30/1 -> _WarnBALLAST/1
  Sammel Error/1 -> Compare To Zero2/1
  RFE Fault/1 -> Compare To Zero17/1
  Compare To Zero22/1 -> _WarnDEVICETEMP/1
  Compare To Zero17/1 -> _RFE FAULT/1
  Data Type Conversion/1 -> BADPARAS/1, RFE Fault/1, BUS TIMEOUT/1, FEEDBACK/1, POWERVOLTAGE/1, MOTORTEMP/1, DEVICETEMP/1, Sammel Error/1, POWER FAULT/1, OVERVOLTAGE/1, RACEAWAY/1, USER/1, I2R/1, HW_FAIL/1, BALLAST/1, I_PEAK/1, WarnWARNING_0/1, WarnILLEGAL_STATUS/1, WarnWARNING_2/1, WarnMOTORTEMP/1, WarnDEVICETEMP/1, Sammel Warnung/1, WarnPOWERVOLTAGE/1, WarnOVERVOLTAGE/1, WarnI_peak/1, WarnI2R/1, WarnBALLAST/1
  I2R/1 -> Compare To Zero12/1
  Compare To Zero21/1 -> _WarnMOTORTEMP/1
  Compare To Zero20/1 -> _WarnPOWERVOLTAGE/1
  Compare To Zero19/1 -> _WarnWARNING_2/1
  Compare To Zero18/1 -> _WarnILLEGAL_STATUS/1
  Compare To Zero24/1 -> _WarnI_peak/1
  WarnILLEGAL_STATUS/1 -> Compare To Zero18/1
  Compare To Zero13/1 -> _WarnWARNING_0/1
  WarnWARNING_2/1 -> Compare To Zero19/1
  WarnWARNING_0/1 -> Compare To Zero13/1

== system DR18E_Testpult/Eingabe Fahrzeug/Inverter Feedback Messages/Istwerte Umrichter 2 empfangen/Sender OK Detection ==
  note: This subsystem implements the surveying of the sender corresponding to the RX message.
      |
      | If for 6 consecutive execution steps no message is received it is considered that the sender is no
      | longer alive or in serious trouble and the 'RX Warn' output is set to 1.
      |
      | Also, the message is expected to be received every 50 ms approximatively. If this condition is not
      | met 6 times consecutively the 'RX Warn' output is set to 1.
  RX status : Inport
  RX delta time : Inport  Port=2
  AND : Logic
  Delta time limit : Constant  Value=0.055
  Delta time limit exceeded : RelationalOperator  RndMeth=Nearest  InputSameDT=on
  Mem{1..5} (5 alike) : Memory
  New data : RelationalOperator  Operator===  RndMeth=Nearest  InputSameDT=on
  New data value : Constant
  No data : RelationalOperator  Operator===  RndMeth=Nearest  InputSameDT=on
  No data value : Constant  Value=0
  OR : Logic  Operator=OR
  Warn : Logic  Inputs=6
  RX Warn : Outport
  wires:
  New data value/1 -> New data/2
  Delta time limit exceeded/1 -> AND/2
  Delta time limit/1 -> Delta time limit exceeded/2
  RX delta time/1 -> Delta time limit exceeded/1
  New data/1 -> AND/1
  AND/1 -> OR/2
  No data value/1 -> No data/2
  No data/1 -> OR/1
  RX status/1 -> No data/1, New data/1
  OR/1 -> Mem1/1, Warn/1
  Mem1/1 -> Mem2/1, Warn/2
  Mem2/1 -> Mem3/1, Warn/3
  Mem3/1 -> Mem4/1, Warn/4
  Warn/1 -> RX Warn/1
  Mem4/1 -> Mem5/1, Warn/5
  Mem5/1 -> Warn/6

== system DR18E_Testpult/Eingabe Fahrzeug/Inverter Feedback Messages/Istwerte Umrichter 2 empfangen/Strom ==
  In2 : Inport
  Action Port : ActionPort  ActionType=case
  Constant2 : Constant  Value=560
  Data Type Conversion3 : DataTypeConversion  OutDataTypeStr=int16
  Divide2 : Product  Inputs=*/
  Drehmoment / Strangstrom in Nm/Arms : Gain  Gain=0.75
  Gain2 : Gain  Gain=200
  Strangstrom I_rms in A U1 : Outport
  Drehmoment M in Nm U1 : Outport  Port=2
  wires:
  In2/1 -> Data Type Conversion3/1
  Gain2/1 -> Divide2/1
  Constant2/1 -> Divide2/2
  Divide2/1 -> Strangstrom I_rms in A U1/1, Drehmoment / Strangstrom in Nm/Arms/1
  Drehmoment / Strangstrom in Nm/Arms/1 -> Drehmoment M in Nm U1/1
  Data Type Conversion3/1 -> Gain2/1

== system DR18E_Testpult/Eingabe Fahrzeug/Inverter Feedback Messages/Istwerte Umrichter 2 empfangen/U_DC ==
  In1 : Inport
  Action Port : ActionPort  ActionType=case
  Umrechnung Register--> Spannung Manual BAMOCAR PG D3 S. 47 : Gain  Gain=1/31.499
  U_DC : Outport
  wires:
  In1/1 -> Umrechnung Register--> Spannung Manual BAMOCAR PG D3 S. 47/1  "Wert"
  Umrechnung Register--> Spannung Manual BAMOCAR PG D3 S. 47/1 -> U_DC/1

== system DR18E_Testpult/Eingabe Fahrzeug/Inverter Feedback Messages/Istwerte Umrichter 2 empfangen/Wirkstrom Iq ==
  In1 : Inport
  Action Port : ActionPort  ActionType=case
  Constant2 : Constant  Value=560
  Data Type Conversion1 : DataTypeConversion  OutDataTypeStr=int16
  Divide2 : Product  Inputs=*/
  Faktor 3/2 : Constant  Value=1.5
  Gain3 : Gain  Gain=200
  Polpaarzahl p : Constant  Value=10
  Product : Product  Inputs=4
  magnertischer Fluß Psi in Vs : Constant  Value=0.053
  Wirkstrom Iq in A U1 : Outport
  Drehmoment in Nm aus Iq U1 : Outport  Port=2
  wires:
  In1/1 -> Data Type Conversion1/1
  Gain3/1 -> Divide2/1
  Constant2/1 -> Divide2/2
  Polpaarzahl p/1 -> Product/2
  Faktor 3/2/1 -> Product/3
  magnertischer Fluß Psi in Vs/1 -> Product/4
  Product/1 -> Drehmoment in Nm aus Iq U1/1
  Data Type Conversion1/1 -> Gain3/1
  Divide2/1 -> Product/1, Wirkstrom Iq in A U1/1

== system DR18E_Testpult/Eingabe Fahrzeug/Lenkwinkelgeber/RX Timeout Detection/Triggered Subsystem ==
  TXStatus : Inport
  Timeout : Inport  Port=2
  Constant : Constant
  Constant1 : Constant  Value=0
  Constant2 : Constant
  Constant3 : Constant  Value=0
  Delay : Delay  DelayLength=1  InitialCondition=0
  Relational Operator : RelationalOperator  Operator=>  OutDataTypeStr=boolean  RndMeth=Nearest
  Sum : Sum  Inputs=|++
  Switch : Switch  Criteria=u2 > Threshold
  Switch1 : Switch  Criteria=u2 > Threshold
  Rampe : Outport
  RX Timeout Error : Outport  Port=2
  wires:
  TXStatus/1 -> Switch/2
  Delay/1 -> Sum/2
  Constant/1 -> Sum/1
  Sum/1 -> Switch/3
  Switch/1 -> Delay/1, Relational Operator/1, Rampe/1
  Constant1/1 -> Switch/1
  Constant2/1 -> Switch1/1
  Constant3/1 -> Switch1/3
  Switch1/1 -> RX Timeout Error/1
  Relational Operator/1 -> Switch1/2
  Timeout/1 -> Relational Operator/2

== system DR18E_Testpult/Eingabe Fahrzeug/MicroAutoBox/AI/FlightRecorder1 ==
  In1 : Inport
  Data Type Conversion : DataTypeConversion
  Gain : Gain
  USB_FLIGHT_REC_BL1 : rtiusbflightreclib/USB_FLIGHT_REC_BL1  VarName=KuehlwasserTemp  DataType=Single  SampleTime=-1  TLCFileName=rtiusbflightrecwrite  Reserved1=[]  Reserved2=[]  Reserved3=[]  Reserved4=[]  DSProperties=struct('RTI',struct('Version',uint32(3),'BlockType',struct('isSLSource',uint8(0),'isSLSink',uint8(1),'isHWSource',uint8(0),'isHWSink',uint8(0),'isSetup',uint8(0),'isInline',uint8(1),'isNonInline',uint8(0),'isInterrupt',uint8(0),'isChannelwise',uint8(0)),'IOBoardType',{{'DSUSB','FLIGHTREC'}},'UnitType','FLIGHTREC','Identifier','WRITE','DialogType','SL','BlockSet','RTIUSBFLIGHTREC','SlaveProcessor','NONE'))  RTIBlockInterface=struct('InputPortsActive',1,'InputPortsWidth',int32(1),'InputPortsDataType',{{'SS_SINGLE'}},'BlockDisplay',{{['Write to\nUSB Flight Recorder'],'center'}},'IconTransparency','off','InitLevel',3,'BlockName',struct('Token',{{'USB_FLIGHT_REC_BL1'}}),'MaskDescription',['Write input to the Flight Recorder. Recorded data can be referenced by the specified variable.'],'SampleTime',{{-1}})  RTIBlockParameters=struct('VarName',{{'KuehlwasserTemp','OFF',[]}},'DataType',{{'Single','OFF',[]}},'SampleTime',{{-1,'OFF',[]}},'TLCFileName',{{'rtiusbflightrecwrite','OFF',[]}})  RTISFcnParameters=struct('VarName','char','DataType','char','SampleTime','double','TLCFileName','char')  RTIBlockParaDefault=struct('VarName','Var1','DataType','Single','SampleTime',-1,'TLCFileName','rtiusbflightrecwrite')
      settings: SourceProductName=dSPACE RTI USB Flight Rec Blockset
  wires:
  Data Type Conversion/1 -> USB_FLIGHT_REC_BL1/1
  In1/1 -> Gain/1
  Gain/1 -> Data Type Conversion/1

== system DR18E_Testpult/Eingabe Fahrzeug/MicroAutoBox/AI/FlightRecorder4 ==
  In1 : Inport
  Data Type Conversion : DataTypeConversion
  Gain : Gain
  USB_FLIGHT_REC_BL1 : rtiusbflightreclib/USB_FLIGHT_REC_BL1  VarName=UBatt_LV  DataType=Single  SampleTime=-1  TLCFileName=rtiusbflightrecwrite  Reserved1=[]  Reserved2=[]  Reserved3=[]  Reserved4=[]  DSProperties=struct('RTI',struct('Version',uint32(3),'BlockType',struct('isSLSource',uint8(0),'isSLSink',uint8(1),'isHWSource',uint8(0),'isHWSink',uint8(0),'isSetup',uint8(0),'isInline',uint8(1),'isNonInline',uint8(0),'isInterrupt',uint8(0),'isChannelwise',uint8(0)),'IOBoardType',{{'DSUSB','FLIGHTREC'}},'UnitType','FLIGHTREC','Identifier','WRITE','DialogType','SL','BlockSet','RTIUSBFLIGHTREC','SlaveProcessor','NONE'))  RTIBlockInterface=struct('InputPortsActive',1,'InputPortsWidth',int32(1),'InputPortsDataType',{{'SS_SINGLE'}},'BlockDisplay',{{['Write to\nUSB Flight Recorder'],'center'}},'IconTransparency','off','InitLevel',3,'BlockName',struct('Token',{{'USB_FLIGHT_REC_BL1'}}),'MaskDescription',['Write input to the Flight Recorder. Recorded data can be referenced by the specified variable.'],'SampleTime',{{-1}})  RTIBlockParameters=struct('VarName',{{'UBatt_LV','OFF',[]}},'DataType',{{'Single','OFF',[]}},'SampleTime',{{-1,'OFF',[]}},'TLCFileName',{{'rtiusbflightrecwrite','OFF',[]}})  RTISFcnParameters=struct('VarName','char','DataType','char','SampleTime','double','TLCFileName','char')  RTIBlockParaDefault=struct('VarName','Var1','DataType','Single','SampleTime',-1,'TLCFileName','rtiusbflightrecwrite')
      settings: SourceProductName=dSPACE RTI USB Flight Rec Blockset
  wires:
  Data Type Conversion/1 -> USB_FLIGHT_REC_BL1/1
  In1/1 -> Gain/1
  Gain/1 -> Data Type Conversion/1

== system DR18E_Testpult/Eingabe Fahrzeug/MicroAutoBox/AI/Umrechnung ADC-Widerstand ==
  ADC : Inport
  Uref[V] : Inport  Port=2
  ADC-R : Fcn  Expr=-491400000/(45200-(8200*u(2)/u(1)))
  Mux : Mux  Inputs=2
  UrefADC : Gain  Gain=5.0
  R : Outport
  wires:
  ADC-R/1 -> R/1
  Mux/1 -> ADC-R/1
  ADC/1 -> UrefADC/1
  Uref[V]/1 -> Mux/2
  UrefADC/1 -> Mux/1

== system DR18E_Testpult/Eingabe Fahrzeug/MicroAutoBox/AI/Umrechnung ADC-Widerstand1 ==
  ADC : Inport
  Uref[V] : Inport  Port=2
  ADC-R : Fcn  Expr=-491400000/(45200-(8200*u(2)/u(1)))
  Mux : Mux  Inputs=2
  UrefADC : Gain  Gain=5.0
  R : Outport
  wires:
  ADC-R/1 -> R/1
  Mux/1 -> ADC-R/1
  ADC/1 -> UrefADC/1
  Uref[V]/1 -> Mux/2
  UrefADC/1 -> Mux/1

== system DR18E_Testpult/Eingabe Fahrzeug/MicroAutoBox/AI/Umrechnung Widerstand - Temperatur NTC ==
  R : Inport
  BETA : Constant  Value=3976
  Divide : Product  Inputs=*/
  Divide1 : Product  Inputs=*/
  Divide2 : Product  Inputs=*/
  KTemp : Constant
  Math Function : Math  Operator=log  SaturateOnIntegerOverflow=on
  PT1 Discrete1 : Subsystem
  Product : Product
  R25 : Constant  Value=10000
  Sum : Sum  Inputs=|+-
  Sum1 : Sum  Inputs=|+-
  T0 : Constant  Value=273.15
  T1 : Constant  Value=298.15
  T2 : Constant
  T25 : Constant  Value=298.15
  TTemp : Constant  Value=0.5
  Temperatur : Outport
  wires:
  R25/1 -> Divide1/1
  R/1 -> Divide1/2
  Divide1/1 -> Math Function/1
  Math Function/1 -> Product/1
  T25/1 -> Divide2/1
  BETA/1 -> Divide2/2
  Divide2/1 -> Product/2
  T1/1 -> Divide/1
  T2/1 -> Sum/1
  Product/1 -> Sum/2
  Sum/1 -> Divide/2
  Divide/1 -> Sum1/1
  T0/1 -> Sum1/2
  TTemp/1 -> PT1 Discrete1/3(T)
  KTemp/1 -> PT1 Discrete1/2(K)
  Sum1/1 -> PT1 Discrete1/1(u)
  PT1 Discrete1/1(y) -> Temperatur/1

== system DR18E_Testpult/Eingabe Fahrzeug/MicroAutoBox/AI/Umrechnung Widerstand - Temperatur NTC1 ==
  R : Inport
  BETA : Constant  Value=3976
  Divide : Product  Inputs=*/
  Divide1 : Product  Inputs=*/
  Divide2 : Product  Inputs=*/
  KTemp : Constant
  Math Function : Math  Operator=log  SaturateOnIntegerOverflow=on
  PT1 Discrete1 : Subsystem
  Product : Product
  R25 : Constant  Value=10000
  Sum : Sum  Inputs=|+-
  Sum1 : Sum  Inputs=|+-
  T0 : Constant  Value=273.15
  T1 : Constant  Value=298.15
  T2 : Constant
  T25 : Constant  Value=298.15
  TTemp : Constant  Value=0.2
  Temperatur : Outport
  wires:
  R25/1 -> Divide1/1
  R/1 -> Divide1/2
  Divide1/1 -> Math Function/1
  Math Function/1 -> Product/1
  T25/1 -> Divide2/1
  BETA/1 -> Divide2/2
  Divide2/1 -> Product/2
  T1/1 -> Divide/1
  T2/1 -> Sum/1
  Product/1 -> Sum/2
  Sum/1 -> Divide/2
  Divide/1 -> Sum1/1
  T0/1 -> Sum1/2
  TTemp/1 -> PT1 Discrete1/3(T)
  KTemp/1 -> PT1 Discrete1/2(K)
  Sum1/1 -> PT1 Discrete1/1(u)
  PT1 Discrete1/1(y) -> Temperatur/1

== system DR18E_Testpult/Eingabe Fahrzeug/Sensorboard Front/RX Timeout Detection/Triggered Subsystem ==
  TXStatus : Inport
  Timeout : Inport  Port=2
  Constant : Constant
  Constant1 : Constant  Value=0
  Constant2 : Constant
  Constant3 : Constant  Value=0
  Delay : Delay  DelayLength=1  InitialCondition=0
  Relational Operator : RelationalOperator  Operator=>  OutDataTypeStr=boolean  RndMeth=Nearest
  Sum : Sum  Inputs=|++
  Switch : Switch  Criteria=u2 > Threshold
  Switch1 : Switch  Criteria=u2 > Threshold
  Rampe : Outport
  RX Timeout Error : Outport  Port=2
  wires:
  TXStatus/1 -> Switch/2
  Delay/1 -> Sum/2
  Constant/1 -> Sum/1
  Sum/1 -> Switch/3
  Switch/1 -> Delay/1, Relational Operator/1, Rampe/1
  Constant1/1 -> Switch/1
  Constant2/1 -> Switch1/1
  Constant3/1 -> Switch1/3
  Switch1/1 -> RX Timeout Error/1
  Relational Operator/1 -> Switch1/2
  Timeout/1 -> Relational Operator/2

== system DR18E_Testpult/Eingabe Fahrzeug/Sensorboard Front/RX Timeout Detection1/Triggered Subsystem ==
  TXStatus : Inport
  Timeout : Inport  Port=2
  Constant : Constant
  Constant1 : Constant  Value=0
  Constant2 : Constant
  Constant3 : Constant  Value=0
  Delay : Delay  DelayLength=1  InitialCondition=0
  Relational Operator : RelationalOperator  Operator=>  OutDataTypeStr=boolean  RndMeth=Nearest
  Sum : Sum  Inputs=|++
  Switch : Switch  Criteria=u2 > Threshold
  Switch1 : Switch  Criteria=u2 > Threshold
  Rampe : Outport
  RX Timeout Error : Outport  Port=2
  wires:
  TXStatus/1 -> Switch/2
  Delay/1 -> Sum/2
  Constant/1 -> Sum/1
  Sum/1 -> Switch/3
  Switch/1 -> Delay/1, Relational Operator/1, Rampe/1
  Constant1/1 -> Switch/1
  Constant2/1 -> Switch1/1
  Constant3/1 -> Switch1/3
  Switch1/1 -> RX Timeout Error/1
  Relational Operator/1 -> Switch1/2
  Timeout/1 -> Relational Operator/2

== system DR18E_Testpult/Eingabe Fahrzeug/Sensorboard Mitte/RX Timeout Detection/Triggered Subsystem ==
  TXStatus : Inport
  Timeout : Inport  Port=2
  Constant : Constant
  Constant1 : Constant  Value=0
  Constant2 : Constant
  Constant3 : Constant  Value=0
  Delay : Delay  DelayLength=1  InitialCondition=0
  Relational Operator : RelationalOperator  Operator=>  OutDataTypeStr=boolean  RndMeth=Nearest
  Sum : Sum  Inputs=|++
  Switch : Switch  Criteria=u2 > Threshold
  Switch1 : Switch  Criteria=u2 > Threshold
  Rampe : Outport
  RX Timeout Error : Outport  Port=2
  wires:
  TXStatus/1 -> Switch/2
  Delay/1 -> Sum/2
  Constant/1 -> Sum/1
  Sum/1 -> Switch/3
  Switch/1 -> Delay/1, Relational Operator/1, Rampe/1
  Constant1/1 -> Switch/1
  Constant2/1 -> Switch1/1
  Constant3/1 -> Switch1/3
  Switch1/1 -> RX Timeout Error/1
  Relational Operator/1 -> Switch1/2
  Timeout/1 -> Relational Operator/2

== system DR18E_Testpult/RTI Data/RTI Data Store/RTI Data Store/RTI Data Store ==
  RTI Data Store : Subsystem  mask(RTI_DATA_STORE){}
      mask help:
      | RTI Data Store Block. This block is used by RTI to store internal model dependent data. Deleting this block will result in data loss.
      |
      | NEVER DELETE, COPY, OR MODIFY THIS BLOCK!
      mask Help:
      | RTI Data Store Block. This block is used by RTI to store internal model dependent data. Deleting this block will result in data loss.
      | 
      | NEVER DELETE, COPY, OR MODIFY THIS BLOCK!
      mask Display: text(0.5, 0.5, ' ', 'HorizontalAlignment', 'center');

== system DR18E_Testpult/Verarbeitung/Bremse/PT1 Discrete2/Subsystem ==
  T : Inport
  Constant : Constant
  Constant2 : Constant
  Divide : Product  Inputs=*/
  Divide1 : Product  Inputs=*/
  Sum : Sum  Inputs=|++
  Weighted Sample Time : SampleTimeMath  TsampMathOp=Ts Only
  T* : Outport
  wires:
  Divide/1 -> T*/1
  Weighted Sample Time/1 -> Divide1/2
  Constant/1 -> Divide/1
  Sum/1 -> Divide/2
  T/1 -> Divide1/1
  Constant2/1 -> Sum/2
  Divide1/1 -> Sum/1
